simulink model "manning_test_merge_nonlinear"  (R2022b)
settings: Solver=VariableStepAuto  StartTime=0.0  StopTime=5*N  RelTol=1e-3
libraries: cstblocks x5
settings Model: Creator=chuan  LastModifiedBy=chuan

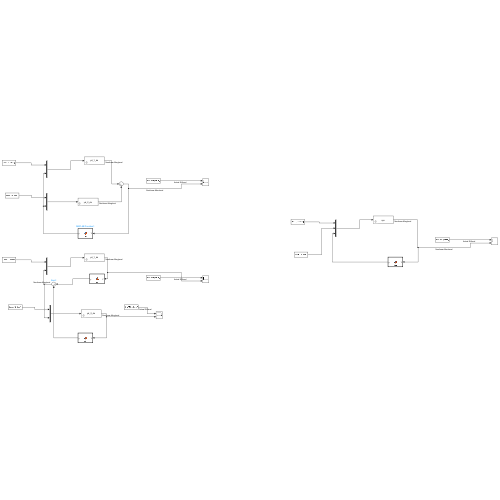
[thumbnail: Simulink's stored preview of the top-level diagram]
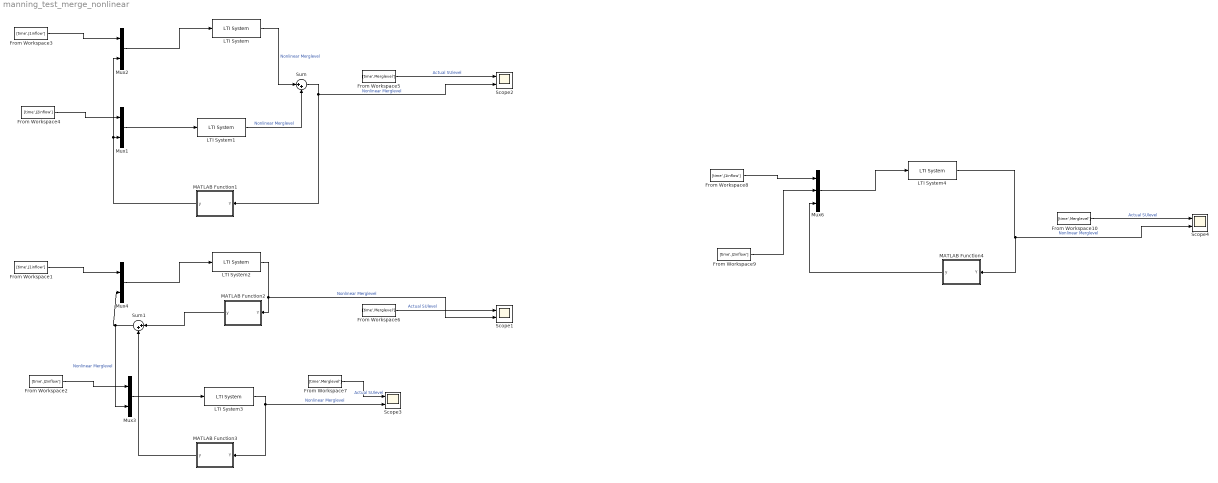
== system manning_test_merge_nonlinear ==
  From Workspace1 : FromWorkspace  VariableName=[time',J1inflow']
  From Workspace{5..7,10} (4 alike) : FromWorkspace  VariableName=[time',Merglevel']
  From Workspace2 : FromWorkspace  VariableName=[time',J2inflow']
  From Workspace3 : FromWorkspace  VariableName=[time',J1inflow']
  From Workspace4 : FromWorkspace  VariableName=[time',J2inflow']
  From Workspace8 : FromWorkspace  VariableName=[time',J1inflow']
  From Workspace9 : FromWorkspace  VariableName=[time',J2inflow']
  LTI System : cstblocks/LTI System  sys=yd_1_ds  IC=[]
  LTI System1 : cstblocks/LTI System  sys=yd_2_ds  IC=[]
  LTI System2 : cstblocks/LTI System  sys=yd_1_ds  IC=[]
  LTI System3 : cstblocks/LTI System  sys=yd_2_ds  IC=[]
  LTI System4 : cstblocks/LTI System  sys=sys  IC=[]
  MATLAB Function1 : MATLAB Function  TreatAsAtomicUnit=on
  MATLAB Function2 : MATLAB Function  TreatAsAtomicUnit=on
  MATLAB Function3 : MATLAB Function  TreatAsAtomicUnit=on
  MATLAB Function4 : MATLAB Function  TreatAsAtomicUnit=on
  Mux{1..4} (4 alike) : Mux  Inputs=2
  Mux6 : Mux  Inputs=3
  Scope{1..4} (4 alike) : Scope  NumInputPorts=2
  Sum : Sum  Inputs=|++
  Sum1 : Sum  Inputs=|++
  wires:
  Mux2/1 -> LTI System/1
  From Workspace5/1 -> Scope2/1  "Actual SUlevel"
  From Workspace3/1 -> Mux2/1
  From Workspace4/1 -> Mux1/1
  Mux1/1 -> LTI System1/1
  LTI System/1 -> Sum/1  "Nonlinear Merglevel"
  LTI System1/1 -> Sum/2  "Nonlinear Merglevel"
  Sum/1 -> MATLAB Function1/1(Y), Scope2/2  "Nonlinear Merglevel"
  MATLAB Function1/1(y) -> Mux2/2, Mux1/2
  From Workspace2/1 -> Mux3/1
  From Workspace6/1 -> Scope1/1  "Actual SUlevel"
  From Workspace1/1 -> Mux4/1
  Mux3/1 -> LTI System3/1
  Mux4/1 -> LTI System2/1
  LTI System2/1 -> Scope1/2, MATLAB Function2/1(Y)  "Nonlinear Merglevel"
  MATLAB Function2/1(y) -> Sum1/1
  LTI System3/1 -> MATLAB Function3/1(Y), Scope3/2  "Nonlinear Merglevel"
  MATLAB Function3/1(y) -> Sum1/2
  Sum1/1 -> Mux3/2, Mux4/2  "Nonlinear Merglevel"
  From Workspace7/1 -> Scope3/1  "Actual SUlevel"
  From Workspace10/1 -> Scope4/1  "Actual SUlevel"
  LTI System4/1 -> MATLAB Function4/1(Y), Scope4/2  "Nonlinear Merglevel"
  From Workspace8/1 -> Mux6/1
  Mux6/1 -> LTI System4/1
  From Workspace9/1 -> Mux6/2
  MATLAB Function4/1(y) -> Mux6/3

== matlab function manning_test_merge_nonlinear/MATLAB Function1 ==
  data: Y input; y output
function y = fcn(Y)
Cd = 0.65;
A0 = 144;
g = 9.81;
Z0 = 1;
Yfull = 12;
H_star = Z0 + Yfull;

Y = max(Y,0);
H1 = Y + Z0;

if H1 >= H_star
    He = H1 - (Z0 + Yfull/2);
    y = Cd*A0*sqrt(2*g*He);
else
    CwL = (Cd*A0*sqrt(g))/(Yfull);
    y = CwL*(H1-Z0)^(1.5);
end

== matlab function manning_test_merge_nonlinear/MATLAB Function3 ==
  data: Y input; y output
function y = fcn(Y)
Cd = 0.65;
A0 = 144;
g = 9.81;
Z0 = 1;
Yfull = 12;
H_star = Z0 + Yfull;

Y = max(Y,0);
H1 = Y + Z0;

if H1 >= H_star
    He = H1 - (Z0 + Yfull/2);
    y = Cd*A0*sqrt(2*g*He);
else
    CwL = (Cd*A0*sqrt(g))/(Yfull);
    y = CwL*(H1-Z0)^(1.5);
end

== matlab function manning_test_merge_nonlinear/MATLAB Function4 ==
  data: Y input; y output
function y = fcn(Y)
Cd = 0.65;
A0 = 144;
g = 9.81;
Z0 = 1;
Yfull = 12;
H_star = Z0 + Yfull;

Y = max(Y,0);
H1 = Y + Z0;

if H1 >= H_star
    He = H1 - (Z0 + Yfull/2);
    y = Cd*A0*sqrt(2*g*He);
else
    CwL = (Cd*A0*sqrt(g))/(Yfull);
    y = CwL*(H1-Z0)^(1.5);
end

== matlab function manning_test_merge_nonlinear/MATLAB Function2 ==
  data: Y input; y output
function y = fcn(Y)
Cd = 0.65;
A0 = 144;
g = 9.81;
Z0 = 1;
Yfull = 12;
H_star = Z0 + Yfull;

Y = max(Y,0);
H1 = Y + Z0;

if H1 >= H_star
    He = H1 - (Z0 + Yfull/2);
    y = Cd*A0*sqrt(2*g*He);
else
    CwL = (Cd*A0*sqrt(g))/(Yfull);
    y = CwL*(H1-Z0)^(1.5);
end
